simulink model "Nonlinear_Simulink"  (R2023b)
settings: Solver=VariableStepAuto  StartTime=0.0  StopTime=10  FixedStep=0.001  RelTol=1e-3
values from neighbouring files (symbols this model uses):
  phi_i = 0    [MPC.m]    (also in Optimal_Trajectory3.mat; Optimal_Trajectory4.mat)
  phip_i = 5    [MPC.m]    (also in Optimal_Trajectory3.mat = 0; Optimal_Trajectory4.mat = 0)
  th_i = 0    [MPC.m]    (also in Optimal_Trajectory3.mat; Optimal_Trajectory4.mat)
  thp_i = 0    [MPC.m]    (also in Optimal_Trajectory3.mat; Optimal_Trajectory4.mat)
libraries: mpclib x1, slpidlib x1
settings Model: Creator=Asus  LastModifiedBy=Asus

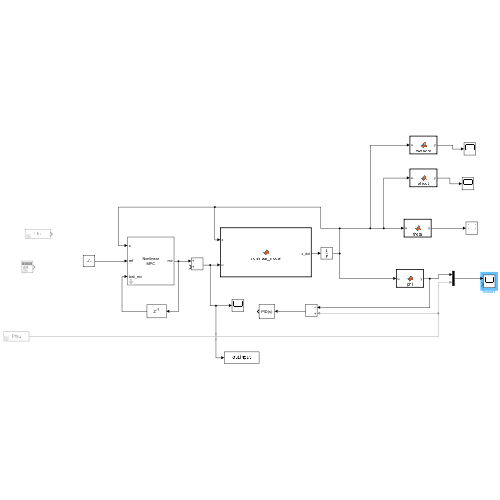
[thumbnail: Simulink's stored preview of the top-level diagram]
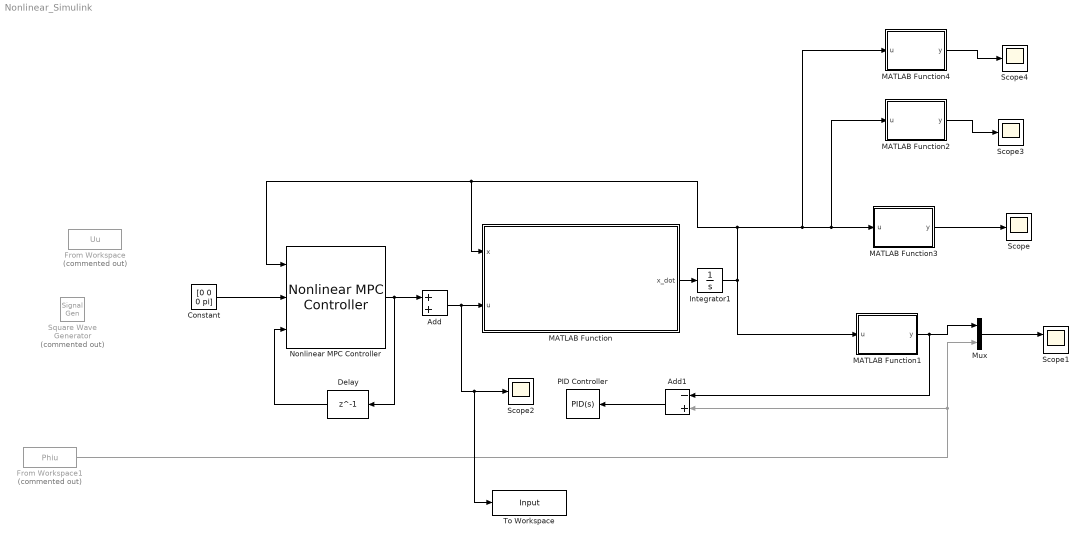
== system Nonlinear_Simulink ==
  Add : Sum
  Add1 : Sum  Inputs=-+
  Constant : Constant  Value=[0 0 0 pi]  VectorParams1D=off
  Delay : Delay  DelayLength=1
  From Workspace : FromWorkspace  Commented=on  VariableName=Uu
  From Workspace1 : FromWorkspace  Commented=on  VariableName=Phiu
  Integrator1 : Integrator  InitialCondition=[thp_i phip_i th_i phi_i]'
  MATLAB Function : MATLAB Function  TreatAsAtomicUnit=on
  MATLAB Function1 : MATLAB Function  TreatAsAtomicUnit=on
  MATLAB Function2 : MATLAB Function  TreatAsAtomicUnit=on
  MATLAB Function3 : MATLAB Function  TreatAsAtomicUnit=on
  MATLAB Function4 : MATLAB Function  TreatAsAtomicUnit=on
  Mux : Mux  Inputs=2
  Nonlinear MPC Controller : mpclib/Nonlinear MPC Controller  nlmpcobj=nlobj  UseObjectTs=on  UseMEX=off  md_enabled=off  mvtarget_enabled=off  param_enabled=off  cost_enabled=off  mvseq_enabled=off  stateseq_enabled=off  ovseq_enabled=off  slack_enabled=off  status_enabled=off  ov_min=off  ov_max=off  mv_min=off  mv_max=off  mvrate_min=off  mvrate_max=off  state_min=off  state_max=off  ov_weight=off  mv_weight=off  mvrate_weight=off  ecr_weight=off  nlp_initialize=off
  PID Controller : slpidlib/PID Controller  Controller=PID  Form=Parallel  TimeDomain=Continuous-time  UseExternalTs=off  SampleTime=-1  IntegratorMethod=Forward Euler  FilterMethod=Forward Euler  ControllerParametersSource=internal  P=30  I=20  UseKiTs=off  D=5  N=100  UseFilter=on  TunerSelectOption=Transfer Function Based (PID Tuner App)  InitialConditionSource=internal  InitialConditionForIntegrator=0  InitialConditionForFilter=0  DifferentiatorICPrevScaledInput=0  ExternalReset=none  TrackingMode=off  Kt=1  LimitOutput=off  SatLimitsSource=internal  UpperSaturationLimit=inf  LowerSaturationLimit=-inf  LinearizeAsGain=on  AntiWindupMode=none  Kb=1  LimitIntegrator=off  UpperIntegratorSaturationLimit=inf  LowerIntegratorSaturationLimit=-inf  POutMin=[]  POutMax=[]  IOutMin=[]  IOutMax=[]  DOutMin=[]  DOutMax=[]  NOutMin=[]  NOutMax=[]  SumOutMin=[]  SumOutMax=[]  SaturationOutMin=[]  SaturationOutMax=[]  PParamMin=[]  PParamMax=[]  IParamMin=[]  IParamMax=[]  DParamMin=[]  DParamMax=[]  NParamMin=[]  NParamMax=[]  KbParamMin=[]  KbParamMax=[]  KtParamMin=[]  KtParamMax=[]  KbOutMin=[]  KbOutMax=[]  KtOutMin=[]  KtOutMax=[]  IntegratorOutMin=[]  IntegratorOutMax=[]  FilterOutMin=[]  FilterOutMax=[]  SumI1OutMin=[]  SumI1OutMax=[]  SumI2OutMin=[]  SumI2OutMax=[]  SumI3OutMin=[]  SumI3OutMax=[]  SumI4OutMin=[]  SumI4OutMax=[]  SumDOutMin=[]  SumDOutMax=[]  DifferentiatorOutMin=[]  DifferentiatorOutMax=[]  FilterDiffOutCoefMin=[]  FilterDiffOutCoefMax=[]  ReciprocalOutMin=[]  ReciprocalOutMax=[]  SumDenOutMin=[]  SumDenOutMax=[]  SumNumOutMin=[]  SumNumOutMax=[]  DivideOutMin=[]  DivideOutMax=[]  UdiffTsProdOutMin=[]  UdiffTsProdOutMax=[]  NTsProdOutMin=[]  NTsProdOutMax=[]  UintegralTsProdOutMin=[]  UintegralTsProdOutMax=[]  UngainTsProdOutMin=[]  UngainTsProdOutMax=[]  ClampingZeroOutDataTypeStr=Inherit: Inherit via back propagation  ClampingZeroOutMin=[]  ClampingZeroOutMax=[]  FilterDenConstantOutDataTypeStr=Inherit: Inherit via back propagation  FilterDenConstantOutMin=[]  FilterDenConstantOutMax=[]  PCopyOutDataTypeStr=Inherit: Inherit via back propagation  PCopyOutMin=[]  PCopyOutMax=[]  NCopyOutDataTypeStr=Inherit: Inherit via back propagation  NCopyOutMin=[]  NCopyOutMax=[]  IntegratorContinuousStateAttributes=''  IntegratorStateMustResolveToSignalObject=off  IntegratorRTWStateStorageClass=Auto  FilterContinuousStateAttributes=''  FilterStateMustResolveToSignalObject=off  FilterRTWStateStorageClass=Auto  ParallelPVariant=InternalParameters  IdealPVariant=Disabled  IVariant=InternalParameters  DVariant=InternalParameters  IntegratorVariant=Continuous  SatVariant=Disabled  AWVariant=Passthrough  PCopyVariant=Disabled  TRVariant=Disabled  FdbkBlocksVariant=Forward  IdealPFdbkVariant=Disabled  SatFdbkVariant=Disabled  DerivativeFilterVariant=ContFilter  NVariant=InternalParameters  NCopyVariant=Disabled  FilterICVariant=InternalICsFilter  IntegratorICVariant=InternalICs  ExternalResetVariant=Disabled  TRSumVariant=Passthrough  SumFdbkVariant=Disabled  SumVariant=Sum_PID  TsampFilterVariant=InternalTs  TsampNgainVariant=Passthrough  TsampIntegralVariant=Disabled_SignalSpec  ExternalSaturationOutDataTypeStr=Inherit: Same as second input
  Scope{,2..4} (4 alike) : Scope
  Scope1 : Scope  NumInputPorts=2
  Square Wave Generator : SignalGenerator  Commented=on  WaveForm=square  Amplitude=5  Frequency=1/0.66  Units=rad/sec
  To Workspace : ToWorkspace  VariableName=Input  SaveFormat=Timeseries  SampleTime=-1
  wires:
  MATLAB Function3/1(y) -> Scope/1
  MATLAB Function4/1(y) -> Scope4/1
  MATLAB Function2/1(y) -> Scope3/1
  From Workspace1/1 -> Mux/2, Add1/2
  Mux/1 -> Scope1/1
  MATLAB Function1/1(y) -> Add1/1, Mux/1
  Integrator1/1 -> MATLAB Function1/1(u), Nonlinear MPC Controller/1, MATLAB Function/1(x), MATLAB Function4/1(u), MATLAB Function2/1(u), MATLAB Function3/1(u)
  MATLAB Function/1(x_dot) -> Integrator1/1
  Add1/1 -> PID Controller/1
  Add/1 -> To Workspace/1, Scope2/1, MATLAB Function/2(u)
  Nonlinear MPC Controller/1 -> Delay/1, Add/1
  Constant/1 -> Nonlinear MPC Controller/2
  Delay/1 -> Nonlinear MPC Controller/3

== matlab function Nonlinear_Simulink/MATLAB Function ==
  data: x input; u input; x_dot output
function x_dot  = nonlinear_model(x,u)


% Arm and Pendulum parameters. 0 for the arm, 1 for the pendulum.
l0 = 0.085; 
l1_tot = 0.12886/2;
l1 = l1_tot-0.0075;
m0 = 0.095;
m1 = 0.024;
% Damping, put here values when measured
d_phi = 2.6173e-06;
d_theta = 0;

% Motor parameters
Jm = 4*10^(-6); %Rotor inertia
kt = 0.042; %Torque constant
Rm = 8.4; %Terminal Resistance
Lm = 1.16*10^(-3); %Rotor Inductance

j0 = m0*l0^2/2 + Jm;
j1 = m1*(l1_tot*2)^2/12;
lx = 0; 
g = 9.81;


% A_1 = [j0+l0^2*m1+l1^2*m1+lx^2*m0-l1^2*m1*cos(x(4))^2, -l0*l1*m1*cos(x(4)),0,0;...
%     -l0*m1*l1*cos(x(4)), m1*l1^2+j1,0,0;0 0 1 0 ;0 0 0 1];
% 
% A_2 = [-l0*l1*m1*sin(x(4))*x(2)^2-2*l1^2*m1*cos(x(4))*sin(x(4))*x(2)*x(1)-kt*kt/Rm*x(1);...
%     m1*cos(x(4))*sin(x(4))*l1^2*x(1)^2-g*m1*sin(x(4))*l1-d_phi*x(2);x(1);x(2)];
% 
% B_1 = [kt/Rm 0 0 0]';
% A = A_1\A_2;
% B = A_1\B_1;
% 
% x_dot = A+B*u;

A_1 = [j0+l0^2*m1+l1^2*m1+lx^2*m0-l1^2*m1*cos(x(4))^2, -l0*l1*m1*cos(x(4)),0,0;...
    -l0*m1*l1*cos(x(4)), m1*l1^2+j1,0,0;0 0 1 0 ;0 0 0 1];

A_2 = [-l0*l1*m1*sin(x(4))*x(2)^2-2*l1^2*m1*cos(x(4))*sin(x(4))*x(2)*x(1)-kt*kt/Rm*x(1);...
    m1*cos(x(4))*sin(x(4))*l1^2*x(1)^2-g*m1*sin(x(4))*l1;x(1);x(2)];

B_1 = u*[kt/Rm 0 0 0]';

A = A_1\A_2;
B = A_1\B_1;

x_dot = A + B;


end

== matlab function Nonlinear_Simulink/MATLAB Function2 ==
  data: u input; y output
function y = phidot(u)

y = u(2);

end

== matlab function Nonlinear_Simulink/MATLAB Function3 ==
  data: u input; y output
function y = theta(u)

y = u(3);

end

== matlab function Nonlinear_Simulink/MATLAB Function4 ==
  data: u input; y output
function y = thetadot(u)

y = u(1);

end

== matlab function Nonlinear_Simulink/MATLAB Function1 ==
  data: u input; y output
function y = phi(u)

y = u(4);

end
